simulink model "Generate_T_Matrix_Boost"  (R2024a)
settings: Solver=ode1be  StartTime=0.0  StopTime=T_end  FixedStep=Ts  RelTol=1e-3  EnableMultiTasking=on
values from neighbouring files (symbols this model uses):
  Ts = 1e-6    (= 1e-06)    [Generate_T_Matrix.m]    (also in Test_T_Matrix.m)
libraries: spsSeriesRLCBranchLib x4, spsCurrentMeasurementLib x3, spsVoltageMeasurementLib x3, spsControlledVoltageSourceLib x2, spsDiodeLib x1, spsGroundLib x1, spsMosfetLib x1, spsPWMGeneratorDCDCLib x1, spspowerguiLib x1
settings Model: Creator=GAO_CX  LastModifiedBy=GAO_CX
settings DataIOCC: SaveOutput=off  SignalLogging=off  DSMLogging=off  SaveTime=off  ReturnWorkspaceOutputs=off
settings ModelReferenceCC: EnableRefExpFcnMdlSchedulingChecks=on
settings RTWCC: GPUComputeCapability=3.5

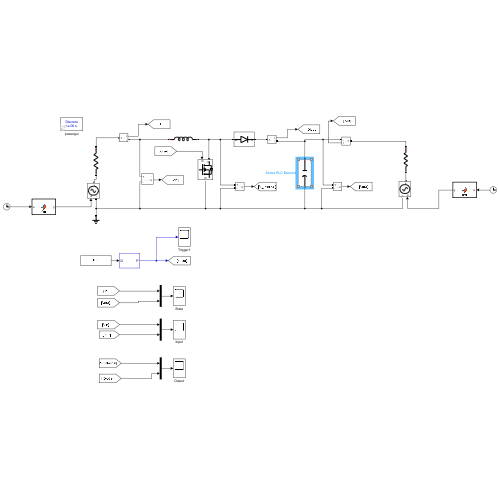
[thumbnail: Simulink's stored preview of the top-level diagram]
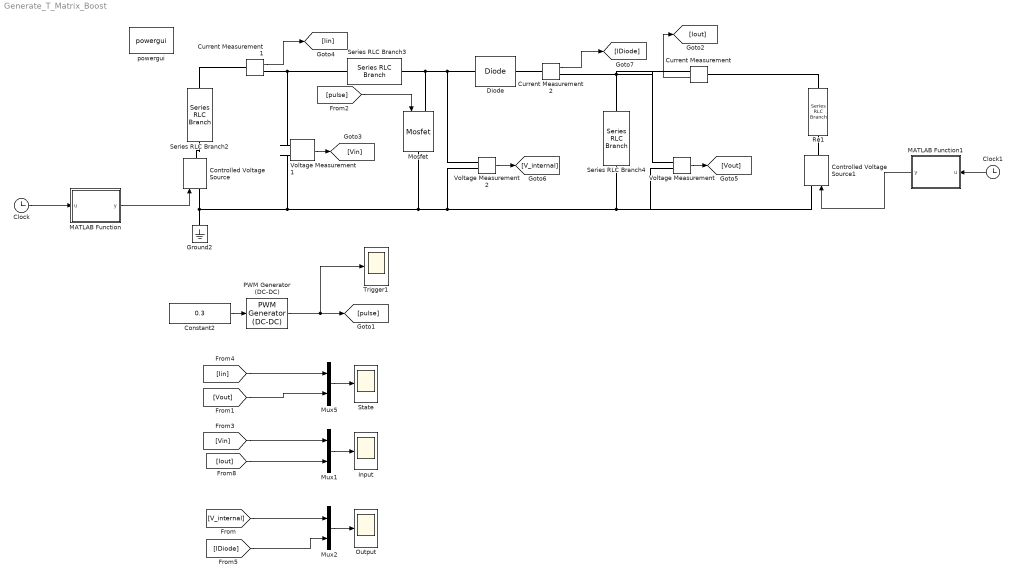
== system Generate_T_Matrix_Boost ==
  Clock : Clock
  Clock1 : Clock
  Constant2 : Constant  Value=0.3
  Controlled Voltage Source : spsControlledVoltageSourceLib/Controlled Voltage Source  Initialize=on  Source_Type=DC  Amplitude=0  Phase=0  Frequency=0  Measurements=None
  Controlled Voltage Source1 : spsControlledVoltageSourceLib/Controlled Voltage Source  Initialize=on  Source_Type=DC  Amplitude=0  Phase=0  Frequency=0  Measurements=None
  Current Measurement : spsCurrentMeasurementLib/Current Measurement  PhasorSimulation=off  OutputType=Complex  PSBequivalent=0
  Current Measurement1 : spsCurrentMeasurementLib/Current Measurement  PhasorSimulation=off  OutputType=Complex  PSBequivalent=0
  Current Measurement2 : spsCurrentMeasurementLib/Current Measurement  PhasorSimulation=off  OutputType=Complex  PSBequivalent=0
  Diode : spsDiodeLib/Diode  Ron=1e-2  Lon=0  Vf=0  IC=0  UseSnubber=0  Rs=inf  Cs=inf  Measurements=off
  Ground2 : spsGroundLib/Ground  LConnTagsString=a
  Input : Scope
  MATLAB Function : MATLAB Function  TreatAsAtomicUnit=on
  MATLAB Function1 : MATLAB Function  TreatAsAtomicUnit=on
  Mosfet : spsMosfetLib/Mosfet  Ron=1e-3  Lon=0  Rd=1e-3  Vfd=0  IC=0  Rs=1e6  Cs=inf  Measurements=off
  Mux1 : Mux  Inputs=2
  Mux2 : Mux  Inputs=2
  Mux5 : Mux  Inputs=2
  Output : Scope
  PWM Generator (DC-DC) : spsPWMGeneratorDCDCLib/PWM Generator (DC-DC)  Fsw=5e3  Ts=0
  Re1 : spsSeriesRLCBranchLib/Series RLC Branch  LConnTagsString=__new0  RConnTagsString=__new0  BranchType=R  Resistance=1  Inductance=1e-3  SetiL0=off  InitialCurrent=0  Capacitance=1e-6  Setx0=off  InitialVoltage=0  Measurements=None
  Series RLC Branch2 : spsSeriesRLCBranchLib/Series RLC Branch  LConnTagsString=__new0  RConnTagsString=__new0  BranchType=R  Resistance=0.01  Inductance=0.04  SetiL0=off  InitialCurrent=0  Capacitance=0.001  Setx0=off  InitialVoltage=0  Measurements=None
  Series RLC Branch3 : spsSeriesRLCBranchLib/Series RLC Branch  LConnTagsString=__new0  RConnTagsString=__new0  BranchType=L  Resistance=0.001  Inductance=1000e-6  SetiL0=off  InitialCurrent=0  Capacitance=0.001  Setx0=off  InitialVoltage=0  Measurements=None
  Series RLC Branch4 : spsSeriesRLCBranchLib/Series RLC Branch  LConnTagsString=__new0  RConnTagsString=__new0  BranchType=C  Resistance=0.001  Inductance=2.5e-2  SetiL0=off  InitialCurrent=0  Capacitance=330e-6  Setx0=off  InitialVoltage=0  Measurements=None
  State : Scope
  Trigger1 : Scope
  Voltage Measurement : spsVoltageMeasurementLib/Voltage Measurement  PhasorSimulation=off  OutputType=Complex  PSBequivalent=0
  Voltage Measurement1 : spsVoltageMeasurementLib/Voltage Measurement  PhasorSimulation=off  OutputType=Complex  PSBequivalent=0
  Voltage Measurement2 : spsVoltageMeasurementLib/Voltage Measurement  PhasorSimulation=off  OutputType=Complex  PSBequivalent=0
  powergui : spspowerguiLib/powergui  Priority=1  SimulationMode=Discrete  SampleTime=Ts  frequency=60  Iterations=50  frequencyindice=0  Pbase=100e6  ErrMax=1e-4  UnitsV=kV  UnitsW=MW  buscounter=0  FunctionMessages=off  echomessages=off  EnableUseOfTLC=off  CurrentSourceSwitches=off  DisableSnubberDevices=off  DisableRonSwitches=off  DisableVfSwitches=off  DisplayEquations=off  AutomaticDiscreteSolvers=off  SolverType=Backward Euler  Interpol=off  ExternalGateDelay=off  methode=off  Ts=0  x0status=blocks  SPID=off  SwTol=0  HookPort=off  NonlinearTolerance=1e-4  nMaxIteration=100  ContinueOnMaxIteration=off  RestoreLinks=warning  ResistiveCurrentMeasurement=off  Frange=[0:2:500]  Ylog=off  Xlog=on  ShowGrid=off  save=off  variable=ZData  structure=0  ZoomFFT=off  StartTime=0.0  cycles=1  DisplayStyle=1  fundamental=60  FreqAxis=off  MaxFrequency=1000  frequencyindicesteady=1  RmsSteady=1  display=off
  wires:
  [Vout] -> Mux5/2
  [Iout] -> Mux1/2
  Voltage Measurement/1 -> [Vout]
  PWM Generator (DC-DC)/1 -> Trigger1/1, [pulse]
  [pulse] -> Mosfet/1
  Current Measurement/1 -> [Iout]
  Voltage Measurement1/1 -> [Vin]
  [Vin] -> Mux1/1
  Current Measurement1/1 -> [Iin]
  [Iin] -> Mux5/1
  Constant2/1 -> PWM Generator (DC-DC)/1
  Mux5/1 -> State/1
  Mux1/1 -> Input/1
  Voltage Measurement2/1 -> [V_internal]
  MATLAB Function/1(y) -> Controlled Voltage Source/1
  Clock/1 -> MATLAB Function/1(u)
  MATLAB Function1/1(y) -> Controlled Voltage Source1/1
  Clock1/1 -> MATLAB Function1/1(u)
  Current Measurement2/1 -> [IDiode]
  [V_internal] -> Mux2/1
  [IDiode] -> Mux2/2
  Mux2/1 -> Output/1
  connections:
  Ground2/LConn1 -- Voltage Measurement1/LConn2 -- Mosfet/RConn1 -- Voltage Measurement2/LConn2 -- Voltage Measurement/LConn2 -- Controlled Voltage Source1/LConn1 -- Series RLC Branch4/RConn1 -- Controlled Voltage Source/LConn1
  Voltage Measurement1/LConn1 -- Series RLC Branch3/LConn1 -- Current Measurement1/RConn1
  Current Measurement/RConn1 -- Voltage Measurement/LConn1 -- Current Measurement2/RConn1 -- Series RLC Branch4/LConn1
  Voltage Measurement2/LConn1 -- Diode/LConn1 -- Mosfet/LConn1 -- Series RLC Branch3/RConn1
  Re1/LConn1 -- Current Measurement/LConn1
  Current Measurement1/LConn1 -- Series RLC Branch2/LConn1
  Series RLC Branch2/RConn1 -- Controlled Voltage Source/RConn1
  Controlled Voltage Source1/RConn1 -- Re1/RConn1
  Diode/RConn1 -- Current Measurement2/LConn1

== matlab function Generate_T_Matrix_Boost/MATLAB Function1 ==
  data: u input; y output
function y = fcn(u)
   y=min(u*(1/0.05),1)+min(u*(0.5*sqrt(2)/0.05),0.5*sqrt(2))*sin(2*pi*50*u+30/180*pi);

== matlab function Generate_T_Matrix_Boost/MATLAB Function ==
  data: u input; y output
function y = fcn(u)
   y=min(u*(2/0.1),2)+min(u*(0.5*sqrt(2)/0.1),0.5*sqrt(2))*sin(2*pi*50*u);
